simulink model "shiyan2_1"  (R2021b)
settings: Solver=FixedStepAuto  StartTime=0.0  StopTime=50  FixedStep=0.001  RelTol=1e-3
libraries: simulink x1
settings Model: Creator=Administrator  LastModifiedBy=Administrator

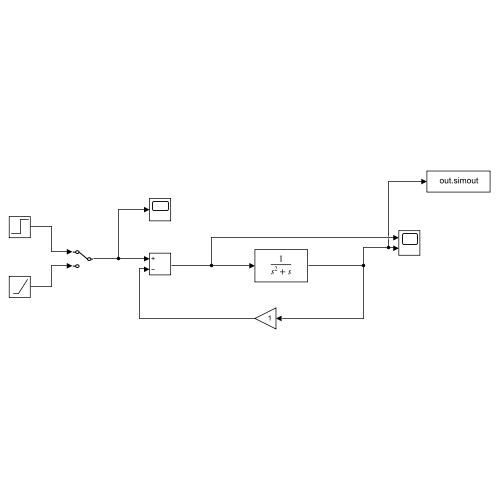
[thumbnail: Simulink's stored preview of the top-level diagram]
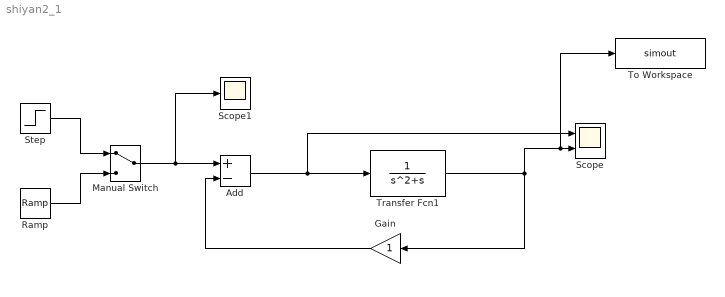
== system shiyan2_1 ==
  Add : Sum  Inputs=+-
  Gain : Gain
  Manual Switch : ManualSwitch
  Ramp : simulink/Sources/Ramp  slope=1  start=0  InitialOutput=0
  Scope : Scope  NumInputPorts=2
  Scope1 : Scope
  Step : Step  Time=0  SampleTime=0
  To Workspace : ToWorkspace  VariableName=simout  SaveFormat=Timeseries  SampleTime=-1
  Transfer Fcn1 : TransferFcn  Denominator=[1 1 0]
  wires:
  Transfer Fcn1/1 -> To Workspace/1, Scope/2, Gain/1
  Gain/1 -> Add/2
  Ramp/1 -> Manual Switch/2
  Manual Switch/1 -> Add/1, Scope1/1
  Step/1 -> Manual Switch/1
  Add/1 -> Scope/1, Transfer Fcn1/1
